simulink model "ICC"  (Simulink 8.4)
settings: Solver=ode45  StartTime=0.0  StopTime=10.0  RelTol=1e-3
undefined symbols (not defined in the file): ICC_atManiOff, ICC_atManiOn
settings Model: Creator=YAL9FE  LastModifiedBy=ric9fe
settings DebuggingCC: FcnCallInpInsideContextMsg=EnableAllAsWarning

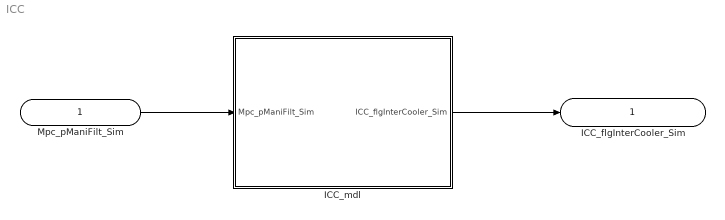
== system ICC ==
  Mpc_pManiFilt_Sim : Inport
  ICC_mdl : Subsystem  mask(Functions){}
      mask help: InterCoolerControl
      mask Display:
      | image(imread('InterCoolerControl.jpg'))
      | port_label('input',1,'Mpc_pManiFilt_Sim')
      | port_label('output',1,'ICC_flgInterCooler_Sim')
  ICC_flgInterCooler_Sim : Outport
  wires:
  Mpc_pManiFilt_Sim/1 -> ICC_mdl/1(Mpc_pManiFilt_Sim)
  ICC_mdl/1(ICC_flgInterCooler_Sim) -> ICC_flgInterCooler_Sim/1

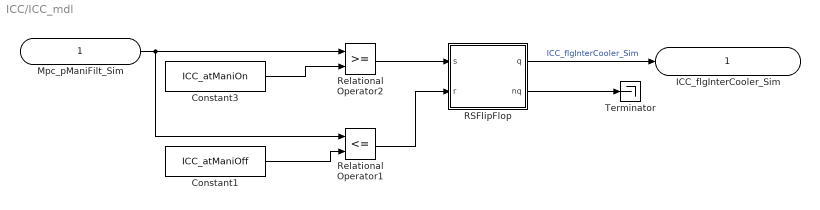
== system ICC/ICC_mdl ==
  Mpc_pManiFilt_Sim : Inport
  Constant1 : Constant  Value=ICC_atManiOff
  Constant3 : Constant  Value=ICC_atManiOn
  RSFlipFlop : Subsystem
      mask help: RSFlipFlop
      mask Display: image(imread('RSFlipFlop.jpg'))
  Relational Operator1 : RelationalOperator  Operator=<=  OutDataTypeStr=boolean
  Relational Operator2 : RelationalOperator  OutDataTypeStr=boolean
  Terminator : Terminator
  ICC_flgInterCooler_Sim : Outport
  wires:
  Mpc_pManiFilt_Sim/1 -> Relational Operator2/1, Relational Operator1/1
  Constant3/1 -> Relational Operator2/2
  Constant1/1 -> Relational Operator1/2
  RSFlipFlop/1(q) -> ICC_flgInterCooler_Sim/1  "ICC_flgInterCooler_Sim"
  RSFlipFlop/2(nq) -> Terminator/1
  Relational Operator2/1 -> RSFlipFlop/1(s)
  Relational Operator1/1 -> RSFlipFlop/2(r)

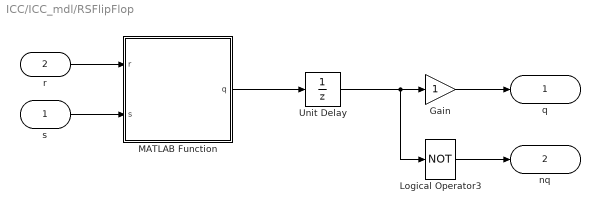
== system ICC/ICC_mdl/RSFlipFlop ==
  s : Inport
  r : Inport  Port=2
  Gain : Gain  OutDataTypeStr=Inherit: Same as input
  Logical Operator3 : Logic  Operator=NOT  AllPortsSameDT=off  OutDataTypeStr=boolean
  MATLAB Function : MATLAB Function  TreatAsAtomicUnit=on
  Unit Delay : UnitDelay  SampleTime=-1
  q : Outport
  nq : Outport  Port=2
  wires:
  Logical Operator3/1 -> nq/1
  r/1 -> MATLAB Function/1(r)
  s/1 -> MATLAB Function/2(s)
  MATLAB Function/1(q) -> Unit Delay/1
  Gain/1 -> q/1
  Unit Delay/1 -> Logical Operator3/1, Gain/1

== matlab function ICC_mdl/RSFlipFlop/MATLAB Function ==
  data: r input double; q output double; s input double
function q = fcn(r,s)
% FlipFlop
q = false;
if(r==true)
    q = false;
elseif(s==true)
    q = true;
end
